simulink library "Saturation_Property"  (Simulink 8.2)
settings: Solver=ode45  StartTime=0.0  StopTime=10.0  RelTol=1e-3
undefined symbols (not defined in the file): CarnotCallbacks_Saturation_Property
settings Model: Creator=lena.frank  LastModifiedBy=drhf

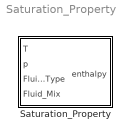
== system Saturation_Property ==
  Saturation_Property : Subsystem  LoadFcn=CarnotCallbacks_Saturation_Property('LoadFcn');  InitFcn=load('THB.mat');  VariantControl=CarlibClassic  mask(saturation property){INPUTARGUMENTS=state variables (classic), PROPERTY=density, FLUIDPHASE=liquid, DEBUGLEVEL=WARNINGLEVEL, MAXTOTALMESSAGES=inf, MAXCONSECUTIVEMESSAGES=inf, WRITETOFILE=0, FILENAME='errors.txt'}
      mask prompts: INPUTARGUMENTS "Input arguments"; FLUIDPHASE "fluid phase"; DEBUGLEVEL "Debug level"; MAXTOTALMESSAGES "maximum number of total warning"; MAXCONSECUTIVEMESSAGES "maximum number of consecutive warnings"; WRITETOFILE "write messages to file"; FILENAME "filename for error messages"
      mask help:
      | The block calculates the saturation value of water by the value of a specified property. Calls the function "saturationproperty" in the CARNOT library "Carlib".
      |
      | PROPERTY            UNIT
      | density                     kg/m³
      | heat capacity           J/kgK
      | heat conductivity     W/mK
      | kinematic viscosity   m²/s
      | enthalpy                   J/kg
      | entropy                     J/kgK
      | prandtl                      --
      | specific volume        m³/kg
      mask init:
      | %Inports
      | CarnotCallbacks_Saturation_Property('CreateInports');
      | 
      | %global debug level
      | [DEBUGLEVEL, MAXTOTALMESSAGES, MAXCONSECUTIVEMESSAGES, WRITETOFILE, FILENAME] = CarnotCallbacks_Saturation_Property('CheckDebugLevels', DEBUGLEVEL, MAXTOTALMESSAGES, MAXCONSECUTIVEMESSAGES, WRITETOFILE, FILENAME);
      mask Help: web(fullfile(path_carnot('help'),'saturationproperty.html'),'-helpbrowser')
      mask TypeOptions INPUTARGUMENTS: state variables (classic) | THB | THV
      mask Callback INPUTARGUMENTS: CarnotCallbacks_Saturation_Property('MaskVisibilities');
      mask TypeOptions PROPERTY: density | heat capacity | heat conductivity | kinematic viscosity | enthalpy | entropy | prandtl | specific volume
      mask TypeOptions FLUIDPHASE: vaporous | liquid | solid
      mask TypeOptions DEBUGLEVEL: DEBUGLEVEL | INFOLEVEL | WARNINGLEVEL | ERRORLEVEL | FATALLEVEL | NOLEVEL

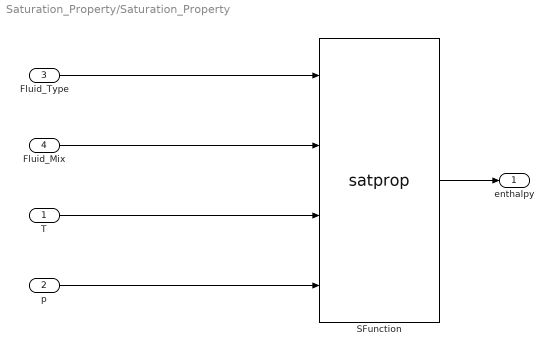
== system Saturation_Property/Saturation_Property ==
  T : Inport
  p : Inport  Port=2
  Fluid_Type : Inport  Port=3
  Fluid_Mix : Inport  Port=4
  SFunction : S-Function  FunctionName=satprop  Parameters=PROPERTY, FLUIDPHASE, DEBUGLEVEL, MAXTOTALMESSAGES, MAXCONSECUTIVEMESSAGES, WRITETOFILE, FILENAME  EnableBusSupport=off
  enthalpy : Outport
  wires:
  SFunction/1 -> enthalpy/1
  T/1 -> SFunction/3
  p/1 -> SFunction/4
  Fluid_Type/1 -> SFunction/1
  Fluid_Mix/1 -> SFunction/2
